simulink model "untitled_2020_before_ACT50_20260612_220843"  (R2024b)
settings: Solver=ode4  StartTime=0  StopTime=15  FixedStep=0.001  RelTol=1e-3
libraries: Solver_SF x1
settings Model: Creator=THY  LastModifiedBy=THY
settings OptimizationCC: DefaultParameterBehavior=Inlined  EnhancedBackFolding=on  PassReuseOutputArgsAs=Individual arguments  ZeroExternalMemoryAtStartup=off  ZeroInternalMemoryAtStartup=off  OptimizeBlockOrder=speed  DifferentSizesBufferReuse=on  OptimizationCustomize=off  EfficientTunableParamExpr=on
settings DebuggingCC: ParameterTunabilityLossMsg=error
settings SFSimCC: MATLABDynamicMemAlloc=off
settings RTWCC: Description=Embedded Coder  SystemTargetFile=ert.tlc  PackageGeneratedCodeAndArtifacts=on  TemplateMakefile=ert_default_tmf
settings CodeAppCC: ForceParamTrailComments=on  IgnoreCustomStorageClasses=off  OperatorAnnotations=on  SimulinkDataObjDesc=on  SFDataObjDesc=on  InsertBlockDesc=on
settings ERTTargetCC: TargetLangStandard=C99 (ISO)  GenerateSampleERTMain=on  SupportContinuousTime=on  SupportNonInlinedSFcns=on  SupportVariableSizeSignals=on  RootIOFormat=Structure reference  ERTCustomFileTemplate=example_file_process.tlc

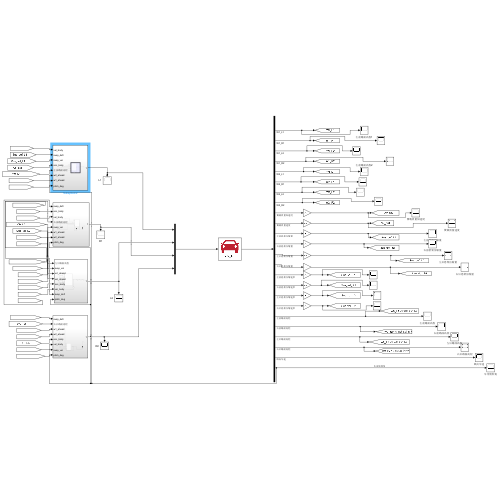
[thumbnail: Simulink's stored preview of the top-level diagram]
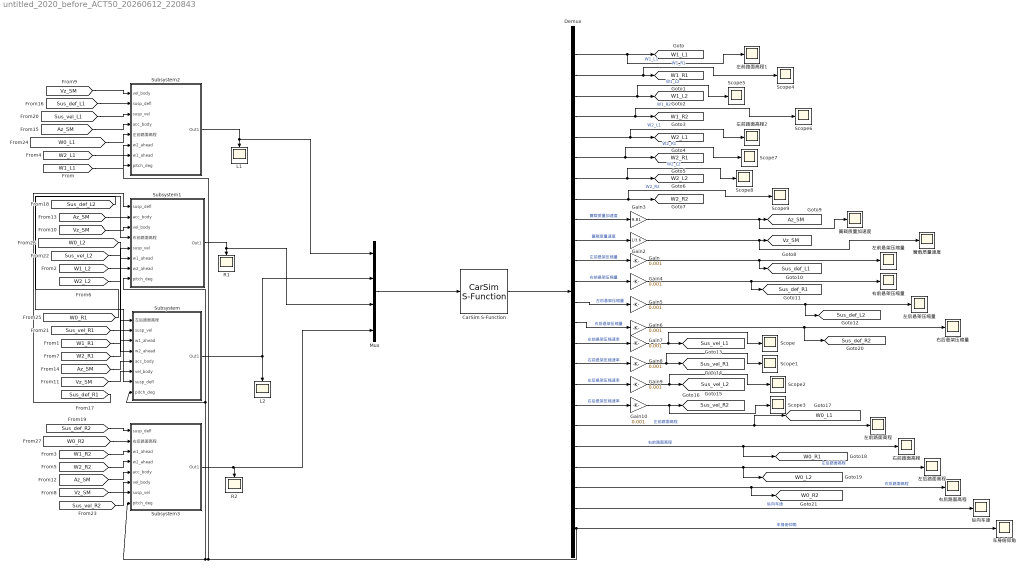
== system untitled_2020_before_ACT50_20260612_220843 ==
  CarSim S-Function : Solver_SF/CarSim S-Function  Priority=1  SIMFILE=simfile.sim  Run_RTs=off  vs_state_ind=Run  StopMode_ind=Vehicle Model
  Demux : Demux  Outputs=24
  Gain{,4..10} (8 alike) : Gain  Gain=0.001
  Gain2 : Gain  Gain=1/3.6
  Gain3 : Gain  Gain=9.81
  L1 : Scope
  L2 : Scope
  Mux : Mux
  R1 : Scope
  R2 : Scope
  Scope{,1..9} (10 alike) : Scope
  Subsystem : Subsystem
  Subsystem1 : Subsystem
  Subsystem2 : Subsystem
  Subsystem3 : Subsystem
  右前悬架压缩量 : Scope
  右前路面高程 : Scope
  右后悬架压缩量 : Scope
  右后路面高程 : Scope
  左前悬架压缩量 : Scope
  左前路面高程 : Scope
  左前路面高程1 : Scope
  左前路面高程2 : Scope
  左后悬架压缩量 : Scope
  左后路面高程 : Scope
  簧载质量加速度 : Scope
  簧载质量速度 : Scope
  纵向车速 : Scope
  车身俯仰角 : Scope
  tag scope: Az_SM=global, Sus_def_L1=global, Sus_def_L2=global, Sus_def_R1=global, Sus_def_R2=global, Sus_vel_L1=global, Sus_vel_L2=global, Sus_vel_R1=global, Sus_vel_R2=global, Vz_SM=global, W0_L1=global, W0_L2=global, W0_R1=global, W0_R2=global, W1_L1=global, W1_L2=global, W1_R1=global, W1_R2=global, W2_L1=global, W2_L2=global, W2_R1=global, W2_R2=global
  wires:
  Subsystem/1(Out1) -> Mux/2, L2/1
  Demux/13 -> Gain5/1  "左后悬架压缩量"
  Demux/11 -> Gain/1  "左前悬架压缩量"
  Demux/9 -> Gain3/1  "簧载质量加速度"
  Demux/23 -> 纵向车速/1  "纵向车速"
  CarSim S-Function/1 -> Demux/1
  Mux/1 -> CarSim S-Function/1
  Subsystem1/1(Out1) -> Mux/3, R1/1
  Gain/1 -> [Sus_def_L1], 左前悬架压缩量/1
  Demux/12 -> Gain4/1  "右前悬架压缩量"
  Demux/10 -> Gain2/1  "簧载质量速度"
  Subsystem2/1(Out1) -> Mux/1, L1/1
  Subsystem3/1(Out1) -> Mux/4, R2/1
  Demux/20 -> [W0_R1], 右前路面高程/1  "右前路面高程"
  Demux/18 -> Gain10/1  "右后悬架压缩速率"
  Demux/16 -> Gain8/1  "右前悬架压缩速率"
  Demux/14 -> Gain6/1  "右后悬架压缩量"
  Demux/19 -> [W0_L1], 左前路面高程/1  "左前路面高程"
  Demux/17 -> Gain9/1  "左后悬架压缩速率"
  Demux/15 -> Gain7/1  "左前悬架压缩速率"
  Demux/24 -> Subsystem/8(pitch_deg), Subsystem1/8(pitch_deg), Subsystem3/8(pitch_deg), Subsystem2/8(pitch_deg), 车身俯仰角/1  "车身俯仰角"
  Demux/22 -> [W0_R2], 右后路面高程/1  "右后路面高程"
  Gain3/1 -> 簧载质量加速度/1, [Az_SM]
  Demux/21 -> [W0_L2], 左后路面高程/1  "左后路面高程"
  Demux/1 -> 左前路面高程1/1, [W1_L1]  "W1_L1"
  Demux/2 -> Scope4/1, [W1_R1]  "W1_R1"
  Demux/3 -> Scope5/1, [W1_L2]  "W1_L2"
  Demux/7 -> Scope8/1, [W2_L2]  "W2_L2"
  Demux/6 -> Scope7/1, [W2_R1]  "W2_R1"
  Demux/5 -> 左前路面高程2/1, [W2_L1]  "W2_L1"
  Demux/4 -> Scope6/1, [W1_R2]  "W1_R2"
  Demux/8 -> Scope9/1, [W2_R2]  "W2_R2"
  [W1_L2] -> Subsystem/3(w1_ahead)
  [W1_R2] -> Subsystem3/3(w1_ahead)
  [W2_L1] -> Subsystem2/6(w2_ahead)
  [W1_L1] -> Subsystem2/7(w1_ahead)
  [W2_R2] -> Subsystem3/4(w2_ahead)
  [W2_L2] -> Subsystem/4(w2_ahead)
  Gain2/1 -> 簧载质量速度/1, [Vz_SM]
  [Vz_SM] -> Subsystem2/1(vel_body)
  [Vz_SM] -> Subsystem3/6(vel_body)
  [Az_SM] -> Subsystem2/4(acc_body)
  [Az_SM] -> Subsystem3/5(acc_body)
  Gain4/1 -> [Sus_def_R1], 右前悬架压缩量/1
  Gain5/1 -> [Sus_def_L2], 左后悬架压缩量/1
  Gain6/1 -> [Sus_def_R2], 右后悬架压缩量/1
  [Sus_def_L1] -> Subsystem2/2(susp_defl)
  Gain7/1 -> Scope/1, [Sus_vel_L1]
  Gain8/1 -> Scope1/1, [Sus_vel_R1]
  Gain9/1 -> Scope2/1, [Sus_vel_L2]
  Gain10/1 -> Scope3/1, [Sus_vel_R2]
  [Sus_def_L2] -> Subsystem/7(susp_defl)
  [Sus_def_R2] -> Subsystem3/1(susp_defl)
  [Sus_vel_L1] -> Subsystem2/3(susp_vel)
  [Sus_vel_L2] -> Subsystem/2(susp_vel)
  [Sus_vel_R2] -> Subsystem3/7(susp_vel)
  [W0_L1] -> Subsystem2/5(左前路面高程)
  [W0_L2] -> Subsystem/1(左后路面高程)
  [W0_R2] -> Subsystem3/2(右后路面高程)
  [Az_SM] -> Subsystem/5(acc_body)
  [Vz_SM] -> Subsystem/6(vel_body)
  [Sus_def_R1] -> Subsystem1/1(susp_defl)
  [Az_SM] -> Subsystem1/2(acc_body)
  [Vz_SM] -> Subsystem1/3(vel_body)
  [W0_R1] -> Subsystem1/4(右前路面高程)
  [Sus_vel_R1] -> Subsystem1/5(susp_vel)
  [W1_R1] -> Subsystem1/6(w1_ahead)
  [W2_R1] -> Subsystem1/7(w2_ahead)

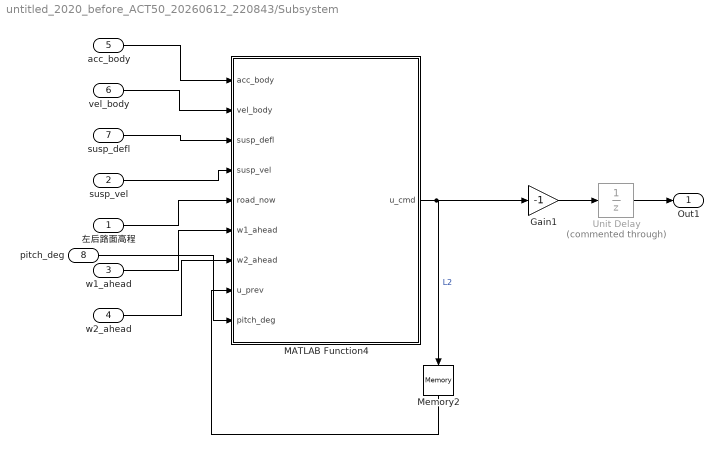
== system untitled_2020_before_ACT50_20260612_220843/Subsystem ==
  左后路面高程 : Inport
  susp_vel : Inport  Port=2
  w1_ahead : Inport  Port=3
  w2_ahead : Inport  Port=4
  acc_body : Inport  Port=5
  vel_body : Inport  Port=6
  susp_defl : Inport  Port=7
  pitch_deg : Inport  Port=8
  Gain1 : Gain  Gain=-1
  MATLAB Function4 : MATLAB Function  TreatAsAtomicUnit=on
  Memory2 : Memory
  Unit Delay : UnitDelay  Commented=through  SampleTime=0.001  HasFrameUpgradeWarning=on
  Out1 : Outport
  wires:
  w2_ahead/1 -> MATLAB Function4/7(w2_ahead)
  susp_defl/1 -> MATLAB Function4/3(susp_defl)
  vel_body/1 -> MATLAB Function4/2(vel_body)
  acc_body/1 -> MATLAB Function4/1(acc_body)
  w1_ahead/1 -> MATLAB Function4/6(w1_ahead)
  左后路面高程/1 -> MATLAB Function4/5(road_now)
  susp_vel/1 -> MATLAB Function4/4(susp_vel)
  Memory2/1 -> MATLAB Function4/8(u_prev)
  MATLAB Function4/1(u_cmd) -> Gain1/1, Memory2/1  "L2"
  Gain1/1 -> Unit Delay/1
  Unit Delay/1 -> Out1/1
  pitch_deg/1 -> MATLAB Function4/9(pitch_deg)

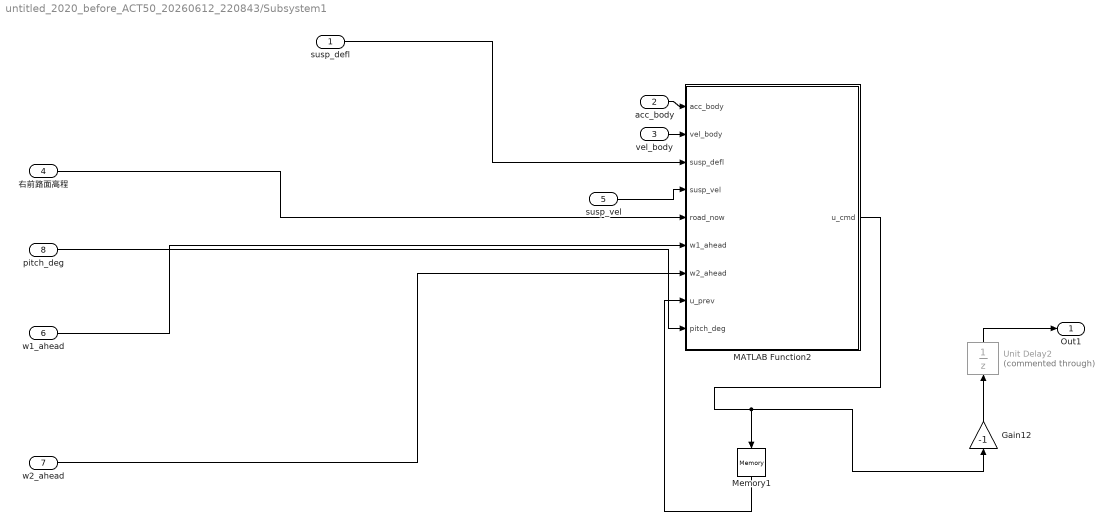
== system untitled_2020_before_ACT50_20260612_220843/Subsystem1 ==
  susp_defl : Inport
  acc_body : Inport  Port=2
  vel_body : Inport  Port=3
  右前路面高程 : Inport  Port=4
  susp_vel : Inport  Port=5
  w1_ahead : Inport  Port=6
  w2_ahead : Inport  Port=7
  pitch_deg : Inport  Port=8
  Gain12 : Gain  Gain=-1
  MATLAB Function2 : MATLAB Function  TreatAsAtomicUnit=on
  Memory1 : Memory  InheritSampleTime=on
  Unit Delay2 : UnitDelay  Commented=through  SampleTime=0.001  HasFrameUpgradeWarning=on
  Out1 : Outport
  wires:
  vel_body/1 -> MATLAB Function2/2(vel_body)
  Unit Delay2/1 -> Out1/1
  Memory1/1 -> MATLAB Function2/8(u_prev)
  Gain12/1 -> Unit Delay2/1
  susp_vel/1 -> MATLAB Function2/4(susp_vel)
  MATLAB Function2/1(u_cmd) -> Memory1/1, Gain12/1
  w1_ahead/1 -> MATLAB Function2/6(w1_ahead)
  右前路面高程/1 -> MATLAB Function2/5(road_now)
  w2_ahead/1 -> MATLAB Function2/7(w2_ahead)
  susp_defl/1 -> MATLAB Function2/3(susp_defl)
  acc_body/1 -> MATLAB Function2/1(acc_body)
  pitch_deg/1 -> MATLAB Function2/9(pitch_deg)

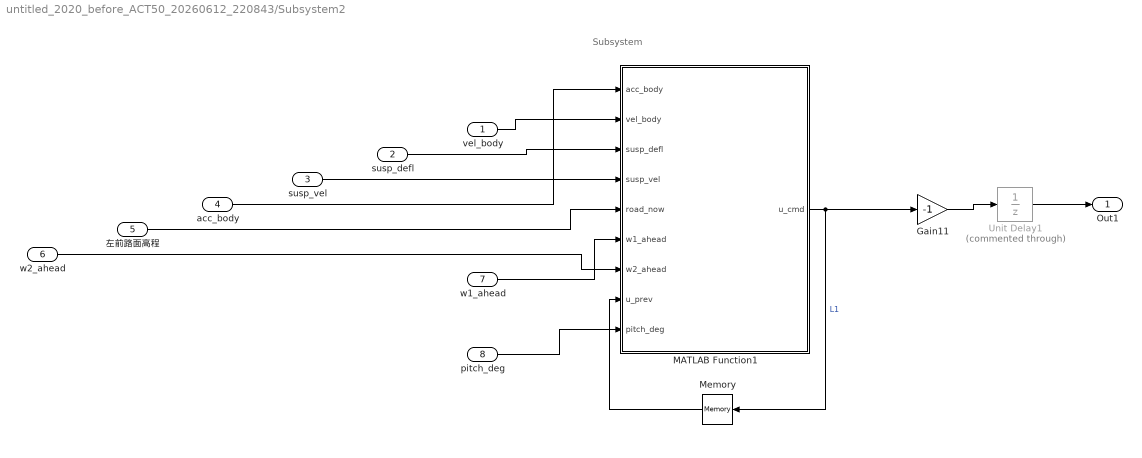
== system untitled_2020_before_ACT50_20260612_220843/Subsystem2 ==
  note: Subsystem
  vel_body : Inport
  susp_defl : Inport  Port=2
  susp_vel : Inport  Port=3
  acc_body : Inport  Port=4
  左前路面高程 : Inport  Port=5
  w2_ahead : Inport  Port=6
  w1_ahead : Inport  Port=7
  pitch_deg : Inport  Port=8
  Gain11 : Gain  Gain=-1
  MATLAB Function1 : MATLAB Function  TreatAsAtomicUnit=on
  Memory : Memory  InheritSampleTime=on
  Unit Delay1 : UnitDelay  Commented=through  SampleTime=0.001  HasFrameUpgradeWarning=on
  Out1 : Outport
  wires:
  Unit Delay1/1 -> Out1/1
  Gain11/1 -> Unit Delay1/1
  pitch_deg/1 -> MATLAB Function1/9(pitch_deg)
  MATLAB Function1/1(u_cmd) -> Gain11/1, Memory/1  "L1"
  w1_ahead/1 -> MATLAB Function1/6(w1_ahead)
  acc_body/1 -> MATLAB Function1/1(acc_body)
  vel_body/1 -> MATLAB Function1/2(vel_body)
  susp_defl/1 -> MATLAB Function1/3(susp_defl)
  susp_vel/1 -> MATLAB Function1/4(susp_vel)
  左前路面高程/1 -> MATLAB Function1/5(road_now)
  w2_ahead/1 -> MATLAB Function1/7(w2_ahead)
  Memory/1 -> MATLAB Function1/8(u_prev)

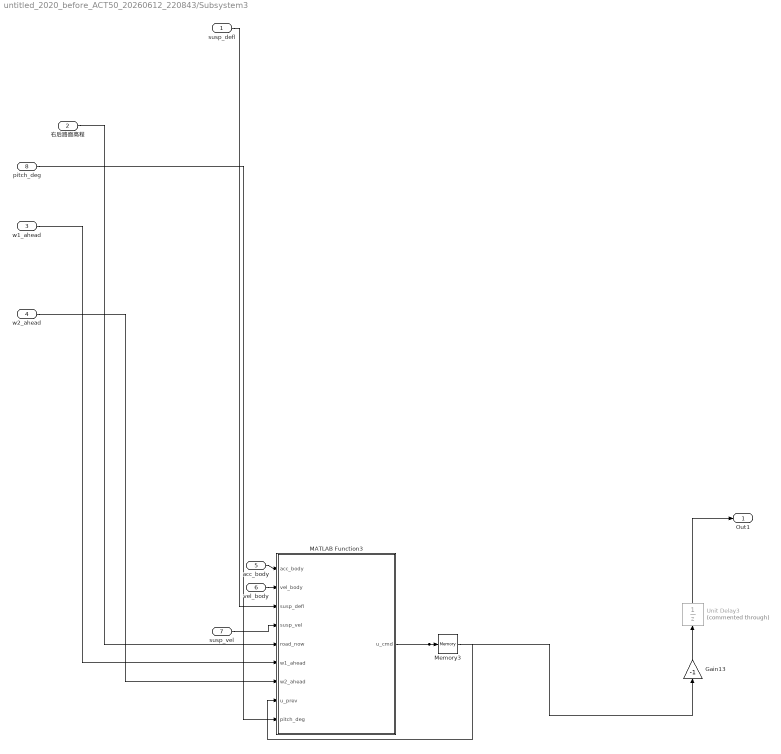
== system untitled_2020_before_ACT50_20260612_220843/Subsystem3 ==
  susp_defl : Inport
  右后路面高程 : Inport  Port=2
  w1_ahead : Inport  Port=3
  w2_ahead : Inport  Port=4
  acc_body : Inport  Port=5
  vel_body : Inport  Port=6
  susp_vel : Inport  Port=7
  pitch_deg : Inport  Port=8
  Gain13 : Gain  Gain=-1
  MATLAB Function3 : MATLAB Function  TreatAsAtomicUnit=on
  Memory3 : Memory
  Unit Delay3 : UnitDelay  Commented=through  SampleTime=0.001  HasFrameUpgradeWarning=on
  Out1 : Outport
  wires:
  w2_ahead/1 -> MATLAB Function3/7(w2_ahead)
  Gain13/1 -> Unit Delay3/1
  Unit Delay3/1 -> Out1/1
  MATLAB Function3/1(u_cmd) -> Memory3/1, Gain13/1
  Memory3/1 -> MATLAB Function3/8(u_prev)
  susp_vel/1 -> MATLAB Function3/4(susp_vel)
  w1_ahead/1 -> MATLAB Function3/6(w1_ahead)
  vel_body/1 -> MATLAB Function3/2(vel_body)
  susp_defl/1 -> MATLAB Function3/3(susp_defl)
  右后路面高程/1 -> MATLAB Function3/5(road_now)
  acc_body/1 -> MATLAB Function3/1(acc_body)
  pitch_deg/1 -> MATLAB Function3/9(pitch_deg)

== matlab function untitled_2020_before_ACT50_20260612_220843/Subsystem2/MATLAB Function1 ==
  data: acc_body input; u_cmd output; vel_body input; susp_defl input; susp_vel input; road_now input; w1_ahead input; w2_ahead input; u_prev input; pitch_deg input
function u_cmd = per_corner_mpc_L1(acc_body, vel_body, susp_defl, susp_vel, road_now, w1_ahead, w2_ahead, u_prev, pitch_deg)
%#codegen
u_cmd = per_corner_mpc_L1_2020(acc_body, vel_body, susp_defl, susp_vel, road_now, w1_ahead, w2_ahead, u_prev, pitch_deg);
end

== matlab function untitled_2020_before_ACT50_20260612_220843/Subsystem1/MATLAB Function2 ==
  data: acc_body input; u_cmd output; vel_body input; susp_defl input; susp_vel input; road_now input; w1_ahead input; w2_ahead input; u_prev input; pitch_deg input
function u_cmd = per_corner_mpc_R1(acc_body, vel_body, susp_defl, susp_vel, road_now, w1_ahead, w2_ahead, u_prev, pitch_deg)
%#codegen
u_cmd = per_corner_mpc_R1_2020(acc_body, vel_body, susp_defl, susp_vel, road_now, w1_ahead, w2_ahead, u_prev, pitch_deg);
end

== matlab function untitled_2020_before_ACT50_20260612_220843/Subsystem3/MATLAB Function3 ==
  data: acc_body input; u_cmd output; vel_body input; susp_defl input; susp_vel input; road_now input; w1_ahead input; w2_ahead input; u_prev input; pitch_deg input
function u_cmd = per_corner_mpc_R2(acc_body, vel_body, susp_defl, susp_vel, road_now, w1_ahead, w2_ahead, u_prev, pitch_deg)
%#codegen
u_cmd = per_corner_mpc_R2_2020(acc_body, vel_body, susp_defl, susp_vel, road_now, w1_ahead, w2_ahead, u_prev, pitch_deg);
end

== matlab function untitled_2020_before_ACT50_20260612_220843/Subsystem/MATLAB Function4 ==
  data: acc_body input; u_cmd output; vel_body input; susp_defl input; susp_vel input; road_now input; w1_ahead input; w2_ahead input; u_prev input; pitch_deg input
function u_cmd = per_corner_mpc_L2(acc_body, vel_body, susp_defl, susp_vel, road_now, w1_ahead, w2_ahead, u_prev, pitch_deg)
%#codegen
u_cmd = per_corner_mpc_L2_2020(acc_body, vel_body, susp_defl, susp_vel, road_now, w1_ahead, w2_ahead, u_prev, pitch_deg);
end
